simulink model "FDA_cosim"  (Simulink 6.6)
settings: Solver=VariableStepDiscrete  StartTime=0.0  StopTime=10  RelTol=1e-3
undefined symbols (not defined in the file): get
libraries: xbsIndex_r4 x7, dspsrcs4 x2, simulink x1, dspsnks4 x1
settings Model: Creator=lcrockett  LastModifiedBy=lcrockett
settings OptimizationCC: InlineParams=on
settings DebuggingCC: SignalResolutionControl=TryResolveAllWithWarning  MultiTaskDSMMsg=warning  MultiTaskCondExecSysMsg=none  StrictBusMsg=None
settings RTWCC: IncludeERTFirstTime=on

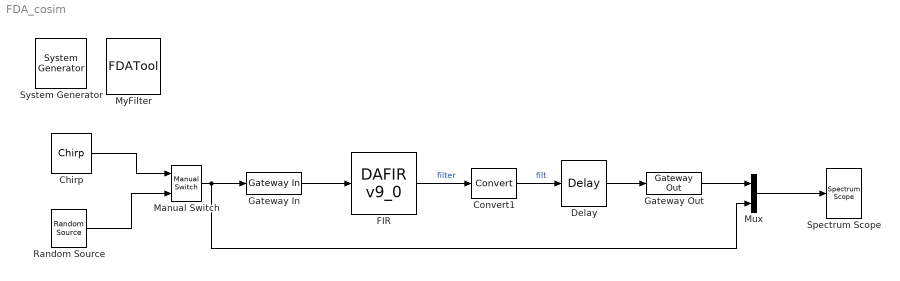
== system FDA_cosim ==
  " System Generator" : xbsIndex_r4/ System Generator  Tag=genX  SystemSampleTime=-1  xilinxfamily=Virtex2P  part=xc2vp30  speed=-7  package=ff896  synthesis_tool=XST  directory=./netlist  testbench=on  simulink_period=1/1.5e6  sysclk_period=67  incr_netlist=off  trim_vbits=Everywhere in SubSystem  dbl_ovrd=According to Block Masks  core_generation=According to Block Masks  run_coregen=off  deprecated_control=off  eval_field=0  block_type=sysgen
      settings: block_version=8.2
  Chirp : dspsrcs4/Chirp  sweep=Swept cosine  mode=Bidirectional  f0=0  f1=750000  t1=0.05  Tsweep=0.5  phase=0  Ts=1/1500000  spf=1  datatype=Double
  Convert1 : xbsIndex_r4/Convert  arith_type="Signed  (2's comp)"  n_bits=8  bin_pt=6  quantization=Truncate  overflow=Wrap  latency=0  dbl_ovrd=off  pipeline=off  block_type=convert
      settings: xl_area=[0, 0, 0, 0, 0, 0, 0]  block_version=VER_STRING_GOES_HERE
  Delay : xbsIndex_r4/Delay  en=off  latency=1  dbl_ovrd=off  reg_retiming=off  block_type=delay
      settings: infoedit=Hardware notes: A delay line is a chain, each link of which is an SRL16 followed by a flip-flop. If register retiming is enabled, the delay line is a chain of flip-flops.  xl_area=[4 8 0 0 0 0 0]  block_version=VER_STRING_GOES_HERE
  FIR : xbsIndex_r4/DAFIR v9_0   coef=[1 -1]  structure=Inferred from Coefficients  coef_n_bits=8  coef_bin_pt=6  over_sample=1  reload=off  valids=off  rst=off  latency=9  num_channels=1  serial_input=off  polyphase_behavior="Single Rate:  sample in - sample out"  dbl_ovrd=off  explicit_period=off  period=1  use_isim=1  block_type=fir
      settings: infoedit="Hardware notes: Implemented using distributed arithmetic (DA).  The hardware over sampling rate determines the degree of parallelism.  A rate of one produces a fully parallel DA filter.  A rate of n (resp., n+1) for an n-bit input signal produces a fully serial implementation for a non-symmetric (resp., symmetric) impulse response.  Intermediate values produce implementations with intermediate levels of parallelism."  xl_area=[0, 0, 0, 0, 0, 0, 0]  block_version=VER_STRING_GOES_HERE
  Gateway In : xbsIndex_r4/Gateway In  arith_type="Signed  (2's comp)"  n_bits=8  bin_pt=6  quantization=Truncate  overflow=Wrap  period=1/1500000  dbl_ovrd=off  timing_constraint=None  locs_specified=off  LOCs={'AG5'}  block_type=gatewayin
      settings: infoedit="Gateway in block.  Converts inputs of type Simulink integer, double and fixed point to  Xilinx fixed point type.<P><P>Hardware notes:  In hardware these blocks become top level input ports."  xl_area=[0, 0, 0, 0, 0, 0, 0]  block_version=VER_STRING_GOES_HERE
  Gateway Out : xbsIndex_r4/Gateway Out  hdl_port=on  timing_constraint=None  locs_specified=off  LOCs={}  block_type=gatewayout
      settings: infoedit="Gateway out block.  Converts Xilinx fixed point inputs into ouputs of type Simulink integer, double, or fixed point.<P><P>Hardware notes:  In hardware these blocks become top level output ports or are discarded, depending on how they are configured."  xl_area=[0, 0, 0, 0, 0, 0, 0]  block_version=VER_STRING_GOES_HERE
  Manual Switch : simulink/Signal Routing/Manual Switch  SystemSampleTime=-1  sw=1  action=0  varsize=off
  Mux : Mux  Inputs=2
  MyFilter : xbsIndex_r4/FDATool  block_type=fdatool
      settings: infoedit=FDATool  block_version=8.2
  Random Source : dspsrcs4/Random Source  SrcType=Uniform  NormMethod=Ziggurat  CltLength=12  MinVal=0  MaxVal=1  MeanVal=0  VarVal=1  RepMode=Not repeatable  rawSeed=1  IsInherit=off  SampMode=Discrete  SampTime=1/1500000  SampFrame=1  DataType=Double  OutComplex=Real
  Spectrum Scope : dspsnks4/Spectrum Scope  DialogController=dspdialog.SpectrumScope  DialogControllerArgs=DataTag3  SystemSampleTime=-1  ScopeProperties=on  Domain=Frequency  HorizSpan=1  UseBuffer=on  BufferSize=512  Overlap=64  inpFftLenInherit=on  FFTlength=512  numAvg=5  DisplayProperties=off  AxisGrid=on  Memory=off  FrameNumber=on  AxisLegend=off  AxisZoom=off  OpenScopeAtSimStart=on  OpenScopeImmediately=off  FigPos=get(0,'defaultfigureposition')  AxisProperties=off  XUnits=Hertz  XRange=[0...Fs/2]  InheritXIncr=off  XIncr=1/1500000  XLabel=Samples  YUnits=dB  YLabel=Magnitude-squared, dB  LineProperties=off  LineColors=[1 0 0]|[0 0 1]  wintypeSpecScope=Hann  RsSpecScope=50  betaSpecScope=5  winsampSpecScope=Periodic
      settings: YMin=-60  YMax=20
  wires:
  FIR/1 -> Convert1/1  "filter"
  Gateway In/1 -> FIR/1
  Convert1/1 -> Delay/1  "filt"
  Chirp/1 -> Manual Switch/1
  Random Source/1 -> Manual Switch/2
  Manual Switch/1 -> Gateway In/1, Mux/2
  Mux/1 -> Spectrum Scope/1
  Gateway Out/1 -> Mux/1
  Delay/1 -> Gateway Out/1
